simulink library "walkingRobotUtils"  (R2024b)
settings: Solver=VariableStepAuto  StartTime=0.0  StopTime=10.0  RelTol=1e-3
undefined symbols (not defined in the file): ankle_servo_kd, ankle_servo_ki, ankle_servo_kp, back_leg_weight, body_weight, deriv_filter_coeff, foot_x, foot_y, foot_z, gravity, half_leg_weight, height_plane, hip_servo_kd, hip_servo_ki, hip_servo_kp, init_angs_L, init_angs_R, init_height, joint_damping, knee_servo_kd, knee_servo_ki, knee_servo_kp, leg_width, lower_leg_length, max_torque, motion_time_constant, motor_constant, motor_inertia, motor_voltage, plane_x, plane_y, plane_z, smiData, torso_height, torso_length, torso_offset_height, torso_offset_length, torso_offset_x, torso_offset_z, torso_width, torso_x, torso_y, torso_z, upper_leg_length, X, Y, Z
libraries: sm_lib x170, nesl_utility x61, $bdroot x51, simulink_extras x40, simulink x27, slpidlib x14, fl_lib x7, ee_lib x3, Multibody_Multiphysics_Lib x1
(part 9 of 9)

== matlab function walkingRobotUtils/Inverse Kinematics (Control Design) ==
  settings: updateMethod=DISCRETE
  data: pos input; angs output; att input; upper_leg_length parameter; lower_leg_length parameter
function angs = invKin(pos, att, upper_leg_length, lower_leg_length)

    % Unpack
    yaw = att(1);
    pitch = att(2);
    roll = att(3);
    x = pos(1);
    y = pos(2);
    z = pos(3);
    
    % Compute the hip angle
    hipRoll = -atan2(y,-z);
    
    % Call symbolic generated function for 2D leg
    zMod = z/cos(hipRoll);
    
    maxMag = 0.1975;
    mag = sqrt(x^2 + zMod^2);
    if sqrt(x^2 + zMod^2) > maxMag
        x = x*maxMag/mag;
        zMod = zMod*maxMag/mag;
    end
    
    theta = legInvKin(upper_leg_length/100,lower_leg_length/100,-x,zMod);
    
    % Address multiple outputs
    if size(theta,1) == 2
       if theta(1,2) < 0
          hipPitch = theta(2,1);
          kneePitch = theta(2,2);
       else
          hipPitch = theta(1,1);
          kneePitch = theta(1,2);
       end
    else
        hipPitch = theta(1);
        kneePitch = theta(2);
    end
    
    % Compensate for torso attitude and set ankle angles
    hipPitch = hipPitch + pitch;
    anklePitch = -kneePitch - hipPitch;
    ankleRoll  = roll - hipRoll;
    
    % Pack
    angs = [ankleRoll; anklePitch; kneePitch; hipRoll; hipPitch];
    
end
